simulink model "Electrical_System_2018b_obfs"  (R2019b)
settings: Solver=VariableStepAuto  StartTime=0.0  StopTime=5  RelTol=1e-3  AbsTol=1e-3  EnableMultiTasking=on
InitFcn:
  | Steady_State_Initialisation;
StopFcn:
  | %sscexplore(simlog);
  | %Logging
undefined symbols (not defined in the file): abrlhklxvp, aexgmhuedq, afmfmjnutg, afpphrjpnc, ahuxbyvruc, alarvljztt, amxnyqmnuw, aodrlwvqie, aolhmuplyq, aqpmguuqkg, auesgwirzl, aurophlnng, awamelrhru, ayfhvxflxn, azxkacuhqc, babszerikg, bawhdqanwq, bevoqecvei, bltjvqbchx, bmqsuewujl, bsmyqjfgnf, btvjbsmnve, bywgxqeadw, bziaduxaer, bzmcmdqocb, bzsvyvetat, ccsjnrbsih, cdvenygxwh, cedkrnslhx, cjheorclzs, cjrdshrtqx, ckhavyhcza, ckxewznhlz, cmrcgyiplk, conenicnws, cqkejbgjnn, csfnuwymhe, cunupkhwbh, cwzfvzuxxh, dcadmadufn, dcfponivnv, ddtrqjrhjn, dfhoxvkqas, dfrhtcwpne, dfvomcagjv, djijwylxea, dnmeqksrrm, dnzewbdkaa, dsqcykyxav, dtswwlttmm, ecumpidjtv, edegaywrct, ejjjsmnejc, eknqnehjdz, emvdetzouf, esxbqkbahr, etnkkbreiq, eunoiiiirw, ewewcuedir, fatkfxdhtc ... (+386)
libraries: fl_lib x802, ee_lib x362, fl_ps_legacy_lib x160, nesl_utility x85
(part 19 of 26)

== system Electrical_System_2018b_obfs/Redacted_1221/Redacted_7996/Redacted_7418/Redacted_4377/Redacted_6082/Redacted_5129 ==
  Redacted_1091 : ee_lib/Passive/Thermal/Thermal Resistor  R=xukkryhjsj K/W  T_specify=off  T_priority=None  T=tqiwxmipjo K  T_nominal_specify=off  T_nominal_unit=K  T_nominal_value=aelkngfktz  Q_specify=off  Q_priority=None  Q=uecypvqdqw W  Q_nominal_specify=off  Q_nominal_unit=W  Q_nominal_value=dfxrifobdg
      settings: SourceProductName=Simscape Electrical  SourceProductBaseCode=PS  InternalSimscapePortConfiguration="{\"Bottom\":[],\"Left\":[{\"id\":\"A\",\"label\":\"A\",\"type\":\"foundation.thermal.thermal\"}],\"Right\":[{\"id\":\"B\",\"label\":\"B\",\"type\":\"foundation.thermal.thermal\"}],\"Top\":[]}"
  Redacted_3516 : fl_lib/Electrical/Electrical Elements/Switch  R_closed=viaptkjwzx Ohm  G_open=spahjfgthv 1/Ohm  Threshold=dnzewbdkaa  i_specify=off  i_priority=None  i=solngxsjde A  i_nominal_specify=off  i_nominal_unit=A  i_nominal_value=kcgnlcicvg  v_specify=off  v_priority=None  v=pvqprocfho V  v_nominal_specify=off  v_nominal_unit=V  v_nominal_value=hvyevfetqr
      settings: SourceProductName=Simscape
  Redacted_4493 : ee_lib/Passive/Thermal/Thermal Resistor  R=vkzgeqezuu K/W  T_specify=off  T_priority=None  T=esxbqkbahr K  T_nominal_specify=off  T_nominal_unit=K  T_nominal_value=kzpyjzolsz  Q_specify=off  Q_priority=None  Q=zidswjyook W  Q_nominal_specify=off  Q_nominal_unit=W  Q_nominal_value=mpaskulynn
      settings: SourceProductName=Simscape Electrical  SourceProductBaseCode=PS  InternalSimscapePortConfiguration="{\"Bottom\":[],\"Left\":[{\"id\":\"A\",\"label\":\"A\",\"type\":\"foundation.thermal.thermal\"}],\"Right\":[{\"id\":\"B\",\"label\":\"B\",\"type\":\"foundation.thermal.thermal\"}],\"Top\":[]}"
  Redacted_5736 : ee_lib/Semiconductors & Converters/Diode  ModelType=scnymfcyan  Vf=usjfqlowdb V  Ron=jptklmkxco Ohm  Goff=ihriznynzt S  prmExp=aymyrnkeyq  I12=sbueuqiyue A  V12=xralefmnmn V  IS=aazejvtdlh A  ec=lidbrydnsj  I1=aanjbxmvih A  V1=csezzhepis V  RS=hlsmvzlbct Ohm  Tmeas=qwpxhludyc degC  N_series=ngscuduecf  N_parallel=mtvctablcr  Rz=kfmndsfqah Ohm  BV=bisvtzzlmp V  C_param=zzuhuqdxbf  CJ=dgdyeqdnad pF  CJ0=vviixrlmuw pF  VJ=erikpjzwum V  Mgrad=idrwctvgka  Vvec=okvogmauev V  Cvec=ltbtlumqgo pF  FC=hutzvqbjst  Q_param=tfxaxdyfov  iRM=mxcantmjiz A  iF=xjldnwmowj A  didt=knlmkgueiv A/us  trr_factor=zjmxnibovs  trr=xbruedlduk ns  Qrr=rqbcaonvzx s*uA  TT=sescozsnne ns  tau=onhgnodkyy ns  T_param=plqnodbxtj  IS_T2=gunyrtbbui A  I1_T2=kbaugpgxig A  V1_T2=pfkhkcpzef V  Tmeas2=tqjznseuwe degC  EG_param=derhodxtrf  EG=puioajbhgt eV  XTI_param=kgeisxvirz  XTI=ttohkaatoo  dBVdT=qouasokgzj V/K  Tdevice=hapcaufila degC  i_specify=off  i_priority=None  i=fhzvmzekzz A  i_nominal_specify=off  i_nominal_unit=A  i_nominal_value=gxbmpayvch  v_specify=off  v_priority=None  v=busuwkvnmf V  v_nominal_specify=off  v_nominal_unit=V  v_nominal_value=mquxmvisyo  i_capacitor_specify=off  i_capacitor_priority=None  i_capacitor=erdhqvbuqo A  i_capacitor_nominal_specify=off  i_capacitor_nominal_unit=A  i_capacitor_nominal_value=rircubgbtn  v_capacitor_specify=off  v_capacitor_priority=None  v_capacitor=ivjksolhtz V  v_capacitor_nominal_specify=off  v_capacitor_nominal_unit=V  v_capacitor_nominal_value=fbdfrcucsm  power_dissipated_specify=off  power_dissipated_priority=None  power_dissipated=kcgakdxjwx W  power_dissipated_nominal_specify=off  power_dissipated_nominal_unit=W  power_dissipated_nominal_value=hmtdzvxlgr  thermal_network_parameterization=ahnuexnajx  Rth=zqvcvxpppv K/W  Rth_Foster=pikijtguhr K/W  thermal_mass_parameterization=ebiijoiwcx  thermal_mass=xdfmtdtgha J/K  thermal_mass_Foster=alrgsxgqtc J/K  thermal_time_constant=vinydwuarm s  thermal_time_constant_Foster=gzkwvsvsmy s  thermal_mass_initial_temperatures=fpaqdrttzj degC
      settings: SourceProductName=Simscape Electrical  InternalSimscapePortConfiguration="{\"Bottom\":[],\"Left\":[{\"id\":\"p\",\"label\":\"\",\"type\":\"foundation.electrical.electrical\"},{\"id\":\"H\",\"label\":\"H\",\"type\":\"foundation.thermal.thermal\"}],\"Right\":[{\"id\":\"n\",\"label\":\"\",\"type\":\"foundation.electrical.electrical\"}],\"Top\":[]}"
  Redacted_5773 : ee_lib/Passive/Thermal/Thermal Resistor  R=pbykuyqcdd K/W  T_specify=off  T_priority=None  T=wxiejlvzgg K  T_nominal_specify=off  T_nominal_unit=K  T_nominal_value=mfkuttxvwe  Q_specify=off  Q_priority=None  Q=dxpebethas W  Q_nominal_specify=off  Q_nominal_unit=W  Q_nominal_value=tsjrjrjwno
      settings: SourceProductName=Simscape Electrical  SourceProductBaseCode=PS  InternalSimscapePortConfiguration="{\"Bottom\":[],\"Left\":[{\"id\":\"A\",\"label\":\"A\",\"type\":\"foundation.thermal.thermal\"}],\"Right\":[{\"id\":\"B\",\"label\":\"B\",\"type\":\"foundation.thermal.thermal\"}],\"Top\":[]}"
  Redacted_7843 : ee_lib/Semiconductors & Converters/Diode  ModelType=vfubjonbyz  Vf=ovhazgcrzk V  Ron=cvrskrmuqj Ohm  Goff=lhhixvbmqc S  prmExp=qjndrrcrwj  I12=gntvzaamtj A  V12=wuwbzbrrpp V  IS=hzdxbkvqke A  ec=lzufgtgbsv  I1=zjffddejik A  V1=ijrimogulp V  RS=ykiqzyljzc Ohm  Tmeas=htzzchmtfv degC  N_series=hvcvcsiwkf  N_parallel=xydvemqmiv  Rz=otkhgvieqq Ohm  BV=vuygfstuny V  C_param=cqqyubkwai  CJ=uoegdangwr pF  CJ0=plaiwchowh pF  VJ=yenohlnnoo V  Mgrad=eruhhyqxpf  Vvec=svfoknpnpk V  Cvec=zqjlotgxpq pF  FC=ortnyuwzrh  Q_param=zdzueyncpy  iRM=pnzdzmfzlv A  iF=jwwiykcvrz A  didt=hhhqlcepyp A/us  trr_factor=rznizglpmy  trr=swvxsytfmb ns  Qrr=rqufmcdvlt s*uA  TT=pecnigvizl ns  tau=ijpnmgbmsc ns  T_param=qpvjlpxidl  IS_T2=vidgyzqclm A  I1_T2=khiphkkgwk A  V1_T2=pizjjevhmz V  Tmeas2=qreuemgwhd degC  EG_param=ancfqgfkip  EG=ktrhgbakxp eV  XTI_param=brbgadfkca  XTI=ygqbsywepo  dBVdT=eqvegiauyi V/K  Tdevice=drlcvrgbtu degC  i_specify=off  i_priority=None  i=cqcsuzhiqx A  i_nominal_specify=off  i_nominal_unit=A  i_nominal_value=xlakfqcnpk  v_specify=off  v_priority=None  v=hictgeopsi V  v_nominal_specify=off  v_nominal_unit=V  v_nominal_value=ughojcypmy  i_capacitor_specify=off  i_capacitor_priority=None  i_capacitor=hpzqydefid A  i_capacitor_nominal_specify=off  i_capacitor_nominal_unit=A  i_capacitor_nominal_value=tcfiupnxkj  v_capacitor_specify=off  v_capacitor_priority=None  v_capacitor=jmshvmneul V  v_capacitor_nominal_specify=off  v_capacitor_nominal_unit=V  v_capacitor_nominal_value=gayfmkqmju  power_dissipated_specify=off  power_dissipated_priority=None  power_dissipated=mgodbrjsas W  power_dissipated_nominal_specify=off  power_dissipated_nominal_unit=W  power_dissipated_nominal_value=fxyfgqyyze  thermal_network_parameterization=fvnzxsjdmp  Rth=wolwfjnjmr K/W  Rth_Foster=qclpxpisnk K/W  thermal_mass_parameterization=gxtwroopga  thermal_mass=inuccawayp J/K  thermal_mass_Foster=fypkvhimoq J/K  thermal_time_constant=rqyvbrsfkk s  thermal_time_constant_Foster=gsviadgrbu s  thermal_mass_initial_temperatures=udushfwxsp degC
      settings: SourceProductName=Simscape Electrical  InternalSimscapePortConfiguration="{\"Bottom\":[],\"Left\":[{\"id\":\"p\",\"label\":\"\",\"type\":\"foundation.electrical.electrical\"},{\"id\":\"H\",\"label\":\"H\",\"type\":\"foundation.thermal.thermal\"}],\"Right\":[{\"id\":\"n\",\"label\":\"\",\"type\":\"foundation.electrical.electrical\"}],\"Top\":[]}"
  Redacted_9825 : fl_lib/Electrical/Electrical Elements/Switch  R_closed=khogqsphcc Ohm  G_open=bnklxlqulg 1/Ohm  Threshold=bzmcmdqocb  i_specify=off  i_priority=None  i=debufxhmtc A  i_nominal_specify=off  i_nominal_unit=A  i_nominal_value=aobdrgvdef  v_specify=off  v_priority=None  v=jvrbptenmb V  v_nominal_specify=off  v_nominal_unit=V  v_nominal_value=ocwrndnqbv
      settings: SourceProductName=Simscape
  Redacted_3870 : PMIOPort  Side=Left
  Redacted_9209 : PMIOPort  Port=2  Side=Left
  Redacted_7831 : PMIOPort  Port=3  Side=Right
  Redacted_499 : PMIOPort  Port=4  Side=Right
  Redacted_8800 : PMIOPort  Port=5  Side=Left
  Redacted_5226 : PMIOPort  Port=6  Side=Right
  connections:
  Redacted_7843/LConn2 -- Redacted_5773/LConn1
  Redacted_4493/RConn1 -- Redacted_8800/RConn1
  Redacted_499/RConn1 -- Redacted_3516/RConn2
  Redacted_9825/RConn1 -- Redacted_3516/RConn1 -- Redacted_5226/RConn1
  Redacted_1091/RConn1 -- Redacted_4493/LConn1 -- Redacted_5773/RConn1
  Redacted_3870/RConn1 -- Redacted_5736/RConn1
  Redacted_5736/LConn1 -- Redacted_9825/LConn1
  Redacted_7831/RConn1 -- Redacted_9825/RConn2
  Redacted_5736/LConn2 -- Redacted_1091/LConn1
  Redacted_7843/RConn1 -- Redacted_3516/LConn1
  Redacted_7843/LConn1 -- Redacted_9209/RConn1

== system Electrical_System_2018b_obfs/Redacted_1221/Redacted_7996/Redacted_7418/Redacted_4377/Redacted_6082/Redacted_538 ==
  Redacted_2474 : ee_lib/Passive/Thermal/Thermal Resistor  R=tlxbhmhcor K/W  T_specify=off  T_priority=None  T=glxcmexbqk K  T_nominal_specify=off  T_nominal_unit=K  T_nominal_value=rodxnpycsn  Q_specify=off  Q_priority=None  Q=qzyewlatml W  Q_nominal_specify=off  Q_nominal_unit=W  Q_nominal_value=gwgijjmpqo
      settings: SourceProductName=Simscape Electrical  SourceProductBaseCode=PS  InternalSimscapePortConfiguration="{\"Bottom\":[],\"Left\":[{\"id\":\"A\",\"label\":\"A\",\"type\":\"foundation.thermal.thermal\"}],\"Right\":[{\"id\":\"B\",\"label\":\"B\",\"type\":\"foundation.thermal.thermal\"}],\"Top\":[]}"
  Redacted_3959 : ee_lib/Semiconductors & Converters/Diode  ModelType=cvugfgmtfd  Vf=orelrxevia V  Ron=wxqqpmaddo Ohm  Goff=dngzjrqfwi S  prmExp=alwaagijeo  I12=ddqlkshwcb A  V12=xrkoiubeyy V  IS=xzqvhkoygc A  ec=mmbccpipxa  I1=ryagswhoik A  V1=yrovtgvtuv V  RS=cqohiqgcgo Ohm  Tmeas=hcgkqnpcsd degC  N_series=dhajyiyagh  N_parallel=twliypcbap  Rz=qwuyngymow Ohm  BV=nknpvrzxhu V  C_param=guvgzkombp  CJ=icairznadf pF  CJ0=mzqqqufhew pF  VJ=clgkkuemkj V  Mgrad=xeknterrpa  Vvec=epolkzdkro V  Cvec=ihzesxymmo pF  FC=renthmlyxq  Q_param=jdcgohbezp  iRM=qomoanohux A  iF=berhrdnhlf A  didt=nmtpqyoydb A/us  trr_factor=ellslhrnwb  trr=iwxktrkdlw ns  Qrr=lvsgqazssj s*uA  TT=djywuxkdvp ns  tau=dsvtaxiwkr ns  T_param=lkgbfzstdy  IS_T2=xxalayentz A  I1_T2=ouhmerbjva A  V1_T2=rsvjknjiop V  Tmeas2=gzwycyriyy degC  EG_param=ufydvnqgur  EG=awpclymgzc eV  XTI_param=hewsmdjtfl  XTI=uikenwfmwu  dBVdT=wnhlxqhthu V/K  Tdevice=oyhmqnvbqo degC  i_specify=off  i_priority=None  i=yuxtxukkqw A  i_nominal_specify=off  i_nominal_unit=A  i_nominal_value=tzdopizgpf  v_specify=off  v_priority=None  v=agbhwyzrpj V  v_nominal_specify=off  v_nominal_unit=V  v_nominal_value=ematotugcl  i_capacitor_specify=off  i_capacitor_priority=None  i_capacitor=xujmcaxirs A  i_capacitor_nominal_specify=off  i_capacitor_nominal_unit=A  i_capacitor_nominal_value=sdffyhujvl  v_capacitor_specify=off  v_capacitor_priority=None  v_capacitor=hxtlnoghbu V  v_capacitor_nominal_specify=off  v_capacitor_nominal_unit=V  v_capacitor_nominal_value=ulxhxpyrnl  power_dissipated_specify=off  power_dissipated_priority=None  power_dissipated=kejtoizjdb W  power_dissipated_nominal_specify=off  power_dissipated_nominal_unit=W  power_dissipated_nominal_value=zqnfawynfr  thermal_network_parameterization=drmprivida  Rth=ehoeehkluw K/W  Rth_Foster=rnfrlrqpxo K/W  thermal_mass_parameterization=qpxdavwohv  thermal_mass=dhvivgsoft J/K  thermal_mass_Foster=bbttosewnp J/K  thermal_time_constant=uruvbjugmy s  thermal_time_constant_Foster=vxxdggnndt s  thermal_mass_initial_temperatures=cxuqjhpxqo degC
      settings: SourceProductName=Simscape Electrical  InternalSimscapePortConfiguration="{\"Bottom\":[],\"Left\":[{\"id\":\"p\",\"label\":\"\",\"type\":\"foundation.electrical.electrical\"},{\"id\":\"H\",\"label\":\"H\",\"type\":\"foundation.thermal.thermal\"}],\"Right\":[{\"id\":\"n\",\"label\":\"\",\"type\":\"foundation.electrical.electrical\"}],\"Top\":[]}"
  Redacted_5204 : ee_lib/Semiconductors & Converters/Diode  ModelType=vhkfbcdxxi  Vf=hwocrhyzln V  Ron=nrejuoqraz Ohm  Goff=xoikkoxmpt S  prmExp=sshdgyqrid  I12=abapcaqksv A  V12=rcfonjwkhk V  IS=uxhycfgjjf A  ec=ccjnesusom  I1=dkqtptmenz A  V1=cwkuodtzyn V  RS=bilkvppmaj Ohm  Tmeas=yoefghiwnx degC  N_series=vbhwyhycfg  N_parallel=nkltgmwizt  Rz=hvsuszjqqa Ohm  BV=fiypzfmfcw V  C_param=oozhdefoba  CJ=sfgabkycgd pF  CJ0=fbfiajzyfi pF  VJ=oqefwzhbwp V  Mgrad=ljxgznyykq  Vvec=byqphrqwso V  Cvec=kiphagckdr pF  FC=cfchcpalde  Q_param=ctajamwbgf  iRM=zyzkgvwrwb A  iF=gzcqjdolru A  didt=ehosyigpsp A/us  trr_factor=yrcmqekjvi  trr=uxqgcepufe ns  Qrr=zdwkgjghcs s*uA  TT=gvqnwlgzwi ns  tau=vcapcgxzee ns  T_param=kdsbtpdywb  IS_T2=dytgzmkhng A  I1_T2=pmcdffsnwx A  V1_T2=yirsozpwmg V  Tmeas2=tadzfoaqtg degC  EG_param=lombnbdzaq  EG=syhamdjlbj eV  XTI_param=ujfmodxdji  XTI=pggidhagfw  dBVdT=jqycxgazic V/K  Tdevice=jamzfbwkuq degC  i_specify=off  i_priority=None  i=yrlsqtdcrj A  i_nominal_specify=off  i_nominal_unit=A  i_nominal_value=xvntcjckiw  v_specify=off  v_priority=None  v=jedxxskqdr V  v_nominal_specify=off  v_nominal_unit=V  v_nominal_value=havzscyyds  i_capacitor_specify=off  i_capacitor_priority=None  i_capacitor=tsjkkrkoym A  i_capacitor_nominal_specify=off  i_capacitor_nominal_unit=A  i_capacitor_nominal_value=gtnybtppoh  v_capacitor_specify=off  v_capacitor_priority=None  v_capacitor=kvzillyxwo V  v_capacitor_nominal_specify=off  v_capacitor_nominal_unit=V  v_capacitor_nominal_value=bigwvzuhqf  power_dissipated_specify=off  power_dissipated_priority=None  power_dissipated=hrgpyhajat W  power_dissipated_nominal_specify=off  power_dissipated_nominal_unit=W  power_dissipated_nominal_value=nzqvcegghq  thermal_network_parameterization=ptsabaosyw  Rth=gmkxekgtcr K/W  Rth_Foster=grktmnwzih K/W  thermal_mass_parameterization=bbnolzopgu  thermal_mass=mdlarzsjrd J/K  thermal_mass_Foster=bznhxpubkn J/K  thermal_time_constant=updbvvrtrk s  thermal_time_constant_Foster=thopflkoks s  thermal_mass_initial_temperatures=cwyiuwsawu degC
      settings: SourceProductName=Simscape Electrical  InternalSimscapePortConfiguration="{\"Bottom\":[],\"Left\":[{\"id\":\"p\",\"label\":\"\",\"type\":\"foundation.electrical.electrical\"},{\"id\":\"H\",\"label\":\"H\",\"type\":\"foundation.thermal.thermal\"}],\"Right\":[{\"id\":\"n\",\"label\":\"\",\"type\":\"foundation.electrical.electrical\"}],\"Top\":[]}"
  Redacted_5866 : ee_lib/Passive/Thermal/Thermal Resistor  R=yowuuinfal K/W  T_specify=off  T_priority=None  T=iyyjqewjxa K  T_nominal_specify=off  T_nominal_unit=K  T_nominal_value=cnwhogxdzi  Q_specify=off  Q_priority=None  Q=xatxitavcu W  Q_nominal_specify=off  Q_nominal_unit=W  Q_nominal_value=lovetezeec
      settings: SourceProductName=Simscape Electrical  SourceProductBaseCode=PS  InternalSimscapePortConfiguration="{\"Bottom\":[],\"Left\":[{\"id\":\"A\",\"label\":\"A\",\"type\":\"foundation.thermal.thermal\"}],\"Right\":[{\"id\":\"B\",\"label\":\"B\",\"type\":\"foundation.thermal.thermal\"}],\"Top\":[]}"
  Redacted_6815 : fl_lib/Electrical/Electrical Elements/Switch  R_closed=gkqjhdadlv Ohm  G_open=gspgtvvlfq 1/Ohm  Threshold=reaxmeylvl  i_specify=off  i_priority=None  i=jkwqanynmu A  i_nominal_specify=off  i_nominal_unit=A  i_nominal_value=retrrtohdd  v_specify=off  v_priority=None  v=bvhvmbtprm V  v_nominal_specify=off  v_nominal_unit=V  v_nominal_value=orfswznhsg
      settings: SourceProductName=Simscape
  Redacted_70 : ee_lib/Passive/Thermal/Thermal Resistor  R=radskbcesf K/W  T_specify=off  T_priority=None  T=pzbxgmpntj K  T_nominal_specify=off  T_nominal_unit=K  T_nominal_value=fxdfehzdjb  Q_specify=off  Q_priority=None  Q=wnpgpngqdb W  Q_nominal_specify=off  Q_nominal_unit=W  Q_nominal_value=mvvrjfvzjw
      settings: SourceProductName=Simscape Electrical  SourceProductBaseCode=PS  InternalSimscapePortConfiguration="{\"Bottom\":[],\"Left\":[{\"id\":\"A\",\"label\":\"A\",\"type\":\"foundation.thermal.thermal\"}],\"Right\":[{\"id\":\"B\",\"label\":\"B\",\"type\":\"foundation.thermal.thermal\"}],\"Top\":[]}"
  Redacted_8610 : fl_lib/Electrical/Electrical Elements/Switch  R_closed=ebbxigazsv Ohm  G_open=bymurvxztv 1/Ohm  Threshold=fatkfxdhtc  i_specify=off  i_priority=None  i=ooxbtdevdj A  i_nominal_specify=off  i_nominal_unit=A  i_nominal_value=vtutgwbqlf  v_specify=off  v_priority=None  v=bphxdwqdvi V  v_nominal_specify=off  v_nominal_unit=V  v_nominal_value=jxgusntfnc
      settings: SourceProductName=Simscape
  Redacted_1520 : PMIOPort  Side=Left
  Redacted_1920 : PMIOPort  Port=2  Side=Left
  Redacted_4965 : PMIOPort  Port=3  Side=Right
  Redacted_6828 : PMIOPort  Port=4  Side=Right
  Redacted_6082 : PMIOPort  Port=5  Side=Left
  Redacted_6905 : PMIOPort  Port=6  Side=Right
  connections:
  Redacted_3959/LConn1 -- Redacted_1920/RConn1
  Redacted_3959/RConn1 -- Redacted_6815/LConn1
  Redacted_5204/LConn2 -- Redacted_2474/LConn1
  Redacted_4965/RConn1 -- Redacted_8610/RConn2
  Redacted_5204/LConn1 -- Redacted_8610/LConn1
  Redacted_1520/RConn1 -- Redacted_5204/RConn1
  Redacted_5866/RConn1 -- Redacted_70/LConn1 -- Redacted_2474/RConn1
  Redacted_6905/RConn1 -- Redacted_6815/RConn1 -- Redacted_8610/RConn1
  Redacted_6828/RConn1 -- Redacted_6815/RConn2
  Redacted_70/RConn1 -- Redacted_6082/RConn1
  Redacted_3959/LConn2 -- Redacted_5866/LConn1

== system Electrical_System_2018b_obfs/Redacted_1221/Redacted_7996/Redacted_7418/Redacted_4377/Redacted_6082/Redacted_5550 ==
  Neutral_Negative : Subsystem  VariantControl=Variant1
  Positive_Neutral : Subsystem  VariantControl=Variant3
  Redacted_2952 : Subsystem  VariantControl=Variant2
  Redacted_6826 : PMIOPort  Side=Left
  Redacted_51 : PMIOPort  Port=2  Side=Left
  Redacted_9515 : PMIOPort  Port=3  Side=Left
  Redacted_375 : PMIOPort  Port=4  Side=Right
  Redacted_6304 : PMIOPort  Port=5  Side=Right

== system Electrical_System_2018b_obfs/Redacted_1221/Redacted_7996/Redacted_7418/Redacted_4377/Redacted_6082/Redacted_5711 ==
  Redacted_1131 : ee_lib/Semiconductors & Converters/Diode  ModelType=sgjcxllrwb  Vf=rezwarhnlc V  Ron=wbzpxlludr Ohm  Goff=tokjykannh S  prmExp=iwsikdclek  I12=ndxpqzjahu A  V12=oyqejwvxul V  IS=mveceiwvha A  ec=uuxcdrnxrh  I1=ofqmoxeuin A  V1=vhypwmzhjp V  RS=kpwjpdopvx Ohm  Tmeas=jbuqxwxids degC  N_series=xhtsnjlbqd  N_parallel=paajnctnwf  Rz=dwqreiwlqp Ohm  BV=yeooqkxzdk V  C_param=fuflydgeqt  CJ=ljpqbdycpo pF  CJ0=jbgrvpposm pF  VJ=ywlmgounuw V  Mgrad=zlqpkihwcd  Vvec=swnlxjsfea V  Cvec=tpransojiq pF  FC=teismtbows  Q_param=kzrgworrpy  iRM=enksfiblxd A  iF=bubyvkprkt A  didt=imidgzdgio A/us  trr_factor=kdehgjmswa  trr=ywtdexwfoq ns  Qrr=dyhowxpurl s*uA  TT=tdrpgsjpmg ns  tau=xwtxyhtqlh ns  T_param=kglbvnzolr  IS_T2=jjkoutammx A  I1_T2=hozxsnrmeo A  V1_T2=ojcyvtfvao V  Tmeas2=uzbilkqbml degC  EG_param=nqysccnfec  EG=ifucnavfam eV  XTI_param=wngxburzzp  XTI=ymmwmtduml  dBVdT=krekrcumku V/K  Tdevice=zrczwfcaxw degC  i_specify=off  i_priority=None  i=jssphwnvvg A  i_nominal_specify=off  i_nominal_unit=A  i_nominal_value=jibhoqemck  v_specify=off  v_priority=None  v=biwmugqnkj V  v_nominal_specify=off  v_nominal_unit=V  v_nominal_value=pllakottju  i_capacitor_specify=off  i_capacitor_priority=None  i_capacitor=gdasqvnftj A  i_capacitor_nominal_specify=off  i_capacitor_nominal_unit=A  i_capacitor_nominal_value=xlxqydjrzg  v_capacitor_specify=off  v_capacitor_priority=None  v_capacitor=jsbomwjeni V  v_capacitor_nominal_specify=off  v_capacitor_nominal_unit=V  v_capacitor_nominal_value=lbbdaqqoij  power_dissipated_specify=off  power_dissipated_priority=None  power_dissipated=ttqksqojpg W  power_dissipated_nominal_specify=off  power_dissipated_nominal_unit=W  power_dissipated_nominal_value=pktukgibmd  thermal_network_parameterization=ukdumittgs  Rth=xarbpsrvuf K/W  Rth_Foster=ehmdrospka K/W  thermal_mass_parameterization=igbepyqptu  thermal_mass=gcqxbhpikq J/K  thermal_mass_Foster=lennybeyrl J/K  thermal_time_constant=cyjedarpes s  thermal_time_constant_Foster=aczvdslxpi s  thermal_mass_initial_temperatures=vndblrhnsn degC
      settings: SourceProductName=Simscape Electrical  InternalSimscapePortConfiguration="{\"Bottom\":[],\"Left\":[{\"id\":\"p\",\"label\":\"\",\"type\":\"foundation.electrical.electrical\"},{\"id\":\"H\",\"label\":\"H\",\"type\":\"foundation.thermal.thermal\"}],\"Right\":[{\"id\":\"n\",\"label\":\"\",\"type\":\"foundation.electrical.electrical\"}],\"Top\":[]}"
  Redacted_2394 : fl_lib/Electrical/Electrical Elements/Switch  R_closed=softcbgoyi Ohm  G_open=mrgmmagxyi 1/Ohm  Threshold=afmfmjnutg  i_specify=off  i_priority=None  i=lmpryftbna A  i_nominal_specify=off  i_nominal_unit=A  i_nominal_value=rlcndthfub  v_specify=off  v_priority=None  v=qfybfotxik V  v_nominal_specify=off  v_nominal_unit=V  v_nominal_value=zyqcuaregq
      settings: SourceProductName=Simscape
  Redacted_3905 : ee_lib/Semiconductors & Converters/Diode  ModelType=nfeveyyrwk  Vf=zoxnipqvrl V  Ron=mtrtbspsae Ohm  Goff=dzrkkqnoys S  prmExp=ievifbrmqp  I12=mmnqlsbltn A  V12=iccotdqbos V  IS=mdvbhccktk A  ec=zvzvjmlaaq  I1=glkqrotric A  V1=yvlqfpnpng V  RS=nzwdscfish Ohm  Tmeas=nqkxyaekrd degC  N_series=nxssfyoknr  N_parallel=bahtqbhcpk  Rz=uddicyycvc Ohm  BV=lpfvklzlry V  C_param=fdmpjfrzqu  CJ=tlkmtlddns pF  CJ0=zlulxxuqkq pF  VJ=ehkmpglgid V  Mgrad=ttbwvlbyhc  Vvec=gsdwthuyom V  Cvec=lrvhhiuttc pF  FC=xzutmjviug  Q_param=qknxtjwyrl  iRM=prfitvseyr A  iF=kpkaitodiu A  didt=atkwyawqox A/us  trr_factor=utxssuipxd  trr=rrnoyzonvo ns  Qrr=dlavsnbofe s*uA  TT=ueprzvgvki ns  tau=jjxthajxlq ns  T_param=iixgioxeoz  IS_T2=wkxqlaxaiv A  I1_T2=zwqouuyrqp A  V1_T2=icvdtwdbib V  Tmeas2=quufchgzgc degC  EG_param=dwtsnaxksr  EG=acnxomkusk eV  XTI_param=vbeyylysip  XTI=xalaivvcmy  dBVdT=kxhlpasngh V/K  Tdevice=gzzizoikgr degC  i_specify=off  i_priority=None  i=tynowkxmpx A  i_nominal_specify=off  i_nominal_unit=A  i_nominal_value=uaygorgksr  v_specify=off  v_priority=None  v=tmrxmeyjrs V  v_nominal_specify=off  v_nominal_unit=V  v_nominal_value=bqcnnfwvrh  i_capacitor_specify=off  i_capacitor_priority=None  i_capacitor=imvbpaeqss A  i_capacitor_nominal_specify=off  i_capacitor_nominal_unit=A  i_capacitor_nominal_value=gybwnvfkmn  v_capacitor_specify=off  v_capacitor_priority=None  v_capacitor=igyzppqxtw V  v_capacitor_nominal_specify=off  v_capacitor_nominal_unit=V  v_capacitor_nominal_value=larocdhkvv  power_dissipated_specify=off  power_dissipated_priority=None  power_dissipated=lnzqmvpzim W  power_dissipated_nominal_specify=off  power_dissipated_nominal_unit=W  power_dissipated_nominal_value=spywrtkhsd  thermal_network_parameterization=hddxfofeyy  Rth=jullxwctpz K/W  Rth_Foster=nvhdmofkhg K/W  thermal_mass_parameterization=mkeqkoxjsc  thermal_mass=sxbbhkgscj J/K  thermal_mass_Foster=ktkpfefkzp J/K  thermal_time_constant=rzzrohaxsq s  thermal_time_constant_Foster=kpaqylfjiw s  thermal_mass_initial_temperatures=jazsdptkag degC
      settings: SourceProductName=Simscape Electrical  InternalSimscapePortConfiguration="{\"Bottom\":[],\"Left\":[{\"id\":\"p\",\"label\":\"\",\"type\":\"foundation.electrical.electrical\"},{\"id\":\"H\",\"label\":\"H\",\"type\":\"foundation.thermal.thermal\"}],\"Right\":[{\"id\":\"n\",\"label\":\"\",\"type\":\"foundation.electrical.electrical\"}],\"Top\":[]}"
  Redacted_5143 : ee_lib/Passive/Thermal/Thermal Resistor  R=ybijqqbkuj K/W  T_specify=off  T_priority=None  T=fxspchliwh K  T_nominal_specify=off  T_nominal_unit=K  T_nominal_value=ppuzbfrerj  Q_specify=off  Q_priority=None  Q=bynsukdflj W  Q_nominal_specify=off  Q_nominal_unit=W  Q_nominal_value=wzgdmbkzup
      settings: SourceProductName=Simscape Electrical  SourceProductBaseCode=PS  InternalSimscapePortConfiguration="{\"Bottom\":[],\"Left\":[{\"id\":\"A\",\"label\":\"A\",\"type\":\"foundation.thermal.thermal\"}],\"Right\":[{\"id\":\"B\",\"label\":\"B\",\"type\":\"foundation.thermal.thermal\"}],\"Top\":[]}"
  Redacted_5618 : fl_lib/Electrical/Electrical Elements/Switch  R_closed=kezykkwcel Ohm  G_open=kohltqvzvt 1/Ohm  Threshold=cdvenygxwh  i_specify=off  i_priority=None  i=hmjtisnfth A  i_nominal_specify=off  i_nominal_unit=A  i_nominal_value=nehnrbwlwu  v_specify=off  v_priority=None  v=yztjetatcm V  v_nominal_specify=off  v_nominal_unit=V  v_nominal_value=mbyxixcoyh
      settings: SourceProductName=Simscape
  Redacted_8133 : ee_lib/Passive/Thermal/Thermal Resistor  R=jumrqxyemk K/W  T_specify=off  T_priority=None  T=ohgunjtfhv K  T_nominal_specify=off  T_nominal_unit=K  T_nominal_value=iyidfkkalr  Q_specify=off  Q_priority=None  Q=paihpxggkf W  Q_nominal_specify=off  Q_nominal_unit=W  Q_nominal_value=epallypmhw
      settings: SourceProductName=Simscape Electrical  SourceProductBaseCode=PS  InternalSimscapePortConfiguration="{\"Bottom\":[],\"Left\":[{\"id\":\"A\",\"label\":\"A\",\"type\":\"foundation.thermal.thermal\"}],\"Right\":[{\"id\":\"B\",\"label\":\"B\",\"type\":\"foundation.thermal.thermal\"}],\"Top\":[]}"
  Redacted_9572 : ee_lib/Passive/Thermal/Thermal Resistor  R=ttoaasuswm K/W  T_specify=off  T_priority=None  T=nnfmlqeyqa K  T_nominal_specify=off  T_nominal_unit=K  T_nominal_value=fhorypsrxc  Q_specify=off  Q_priority=None  Q=ckuzftrrgq W  Q_nominal_specify=off  Q_nominal_unit=W  Q_nominal_value=fqmdqwvrwk
      settings: SourceProductName=Simscape Electrical  SourceProductBaseCode=PS  InternalSimscapePortConfiguration="{\"Bottom\":[],\"Left\":[{\"id\":\"A\",\"label\":\"A\",\"type\":\"foundation.thermal.thermal\"}],\"Right\":[{\"id\":\"B\",\"label\":\"B\",\"type\":\"foundation.thermal.thermal\"}],\"Top\":[]}"
  Redacted_4950 : PMIOPort  Side=Left
  Redacted_5258 : PMIOPort  Port=2  Side=Left
  Redacted_5892 : PMIOPort  Port=3  Side=Right
  Redacted_8207 : PMIOPort  Port=4  Side=Right
  Redacted_4180 : PMIOPort  Port=5  Side=Left
  Redacted_8951 : PMIOPort  Port=6  Side=Right
  connections:
  Redacted_3905/LConn2 -- Redacted_8133/LConn1
  Redacted_9572/RConn1 -- Redacted_4180/RConn1
  Redacted_8207/RConn1 -- Redacted_2394/RConn2
  Redacted_5618/RConn1 -- Redacted_2394/RConn1 -- Redacted_8951/RConn1
  Redacted_5143/RConn1 -- Redacted_9572/LConn1 -- Redacted_8133/RConn1
  Redacted_4950/RConn1 -- Redacted_1131/RConn1
  Redacted_1131/LConn1 -- Redacted_5618/LConn1
  Redacted_5892/RConn1 -- Redacted_5618/RConn2
  Redacted_1131/LConn2 -- Redacted_5143/LConn1
  Redacted_3905/RConn1 -- Redacted_2394/LConn1
  Redacted_3905/LConn1 -- Redacted_5258/RConn1

== system Electrical_System_2018b_obfs/Redacted_1221/Redacted_7996/Redacted_7418/Redacted_4377/Redacted_6082/Redacted_5713 ==
  Neutral_Negative : Subsystem  VariantControl=Variant1
  Positive_Neutral : Subsystem  VariantControl=Variant3
  Redacted_1184 : Subsystem  VariantControl=Variant2
  Redacted_6138 : PMIOPort  Side=Left
  Redacted_1431 : PMIOPort  Port=2  Side=Left
  Redacted_7946 : PMIOPort  Port=3  Side=Left
  Redacted_819 : PMIOPort  Port=4  Side=Right
  Redacted_4816 : PMIOPort  Port=5  Side=Right

== system Electrical_System_2018b_obfs/Redacted_1221/Redacted_7996/Redacted_7418/Redacted_4377/Redacted_6082/Redacted_5976 ==
  Neutral_Negative : Subsystem  VariantControl=Variant1
  Positive_Neutral : Subsystem  VariantControl=Variant3
  Redacted_5620 : Subsystem  VariantControl=Variant2
  Redacted_9241 : PMIOPort  Side=Left
  Redacted_5276 : PMIOPort  Port=2  Side=Left
  Redacted_2400 : PMIOPort  Port=3  Side=Left
  Redacted_5406 : PMIOPort  Port=4  Side=Right
  Redacted_1074 : PMIOPort  Port=5  Side=Right

== system Electrical_System_2018b_obfs/Redacted_1221/Redacted_7996/Redacted_7418/Redacted_4377/Redacted_6082/Redacted_6424 ==
  Neutral_Negative : Subsystem  VariantControl=Variant1
  Positive_Neutral : Subsystem  VariantControl=Variant3
  Redacted_7805 : Subsystem  VariantControl=Variant2
  Redacted_4582 : PMIOPort  Side=Left
  Redacted_1544 : PMIOPort  Port=2  Side=Left
  Redacted_1581 : PMIOPort  Port=3  Side=Left
  Redacted_1961 : PMIOPort  Port=4  Side=Right
  Redacted_7479 : PMIOPort  Port=5  Side=Right

== system Electrical_System_2018b_obfs/Redacted_1221/Redacted_7996/Redacted_7418/Redacted_4377/Redacted_6082/Redacted_6448 ==
  Redacted_2500 : ee_lib/Semiconductors & Converters/Diode  ModelType=efectnzfzk  Vf=jxmepmeowj V  Ron=qgxsnpyvap Ohm  Goff=yoppabgzkl S  prmExp=ubpcccmurz  I12=remshksgqe A  V12=lfyuowwnsp V  IS=kniawzssyt A  ec=shjfprvpho  I1=bqvkznozbx A  V1=kanhzjgbwy V  RS=xqskwtorcu Ohm  Tmeas=wkndwwjeju degC  N_series=oemgleyaog  N_parallel=rmwesacawc  Rz=uupgbnboph Ohm  BV=jmlshjudem V  C_param=ejznuqydbf  CJ=jnyvftnijl pF  CJ0=eocfcshsjc pF  VJ=rcqumjutus V  Mgrad=bpwyttzsav  Vvec=xmbkulzqwe V  Cvec=eqgbafiqja pF  FC=fzcbcscgmr  Q_param=hevnohlimn  iRM=fkisxhzojn A  iF=aecufenajy A  didt=wqayegsgya A/us  trr_factor=tyozkzrsye  trr=byygrqxzxs ns  Qrr=ecsprgxdxa s*uA  TT=estselsvjb ns  tau=lnvjuifvwe ns  T_param=jrnxklcvyp  IS_T2=pegzeyggnh A  I1_T2=dfmjfojaum A  V1_T2=dkkcmajvzi V  Tmeas2=mhkasfkmys degC  EG_param=agwssckltu  EG=rfaarmrbja eV  XTI_param=uxzupvrblg  XTI=ospysejegc  dBVdT=tootsfdmyr V/K  Tdevice=kzpnsiiwfr degC  i_specify=off  i_priority=None  i=eihvzvfrzd A  i_nominal_specify=off  i_nominal_unit=A  i_nominal_value=qmmhrurogd  v_specify=off  v_priority=None  v=hizlbruxfz V  v_nominal_specify=off  v_nominal_unit=V  v_nominal_value=ycpyizpqai  i_capacitor_specify=off  i_capacitor_priority=None  i_capacitor=zppifvcjba A  i_capacitor_nominal_specify=off  i_capacitor_nominal_unit=A  i_capacitor_nominal_value=fpmjfabdfd  v_capacitor_specify=off  v_capacitor_priority=None  v_capacitor=stollmyrll V  v_capacitor_nominal_specify=off  v_capacitor_nominal_unit=V  v_capacitor_nominal_value=kndonlhkoo  power_dissipated_specify=off  power_dissipated_priority=None  power_dissipated=btdavdcdiv W  power_dissipated_nominal_specify=off  power_dissipated_nominal_unit=W  power_dissipated_nominal_value=tkklgbzblp  thermal_network_parameterization=bljrklmcju  Rth=xhsqylwmob K/W  Rth_Foster=optpcutsoi K/W  thermal_mass_parameterization=ugcqtdtype  thermal_mass=jsyutsyost J/K  thermal_mass_Foster=twrmylwkjc J/K  thermal_time_constant=xnykkposzd s  thermal_time_constant_Foster=foiqukjmop s  thermal_mass_initial_temperatures=upiyseqegs degC
      settings: SourceProductName=Simscape Electrical  InternalSimscapePortConfiguration="{\"Bottom\":[],\"Left\":[{\"id\":\"p\",\"label\":\"\",\"type\":\"foundation.electrical.electrical\"},{\"id\":\"H\",\"label\":\"H\",\"type\":\"foundation.thermal.thermal\"}],\"Right\":[{\"id\":\"n\",\"label\":\"\",\"type\":\"foundation.electrical.electrical\"}],\"Top\":[]}"
  Redacted_359 : ee_lib/Semiconductors & Converters/Diode  ModelType=scvaiquffk  Vf=gurupglfta V  Ron=ftlaqddzvo Ohm  Goff=sbgfdffxay S  prmExp=ukcnmjtiae  I12=grbxogokac A  V12=wmzyrlvpsn V  IS=leyegtjcol A  ec=lwvjfwcdkf  I1=dljtokvayx A  V1=irawojoicp V  RS=axoqkcbxfn Ohm  Tmeas=aargryzkwo degC  N_series=kaksezvljy  N_parallel=xdnjyjftou  Rz=rcunxliptk Ohm  BV=hrrjansjso V  C_param=gklskhmoru  CJ=imyuobqtwk pF  CJ0=ewdqrpecjy pF  VJ=wfjksexohd V  Mgrad=jgqtcmmwqv  Vvec=aguvzvrglj V  Cvec=zssvjevjde pF  FC=oeclxcixjt  Q_param=xrpxrrdafl  iRM=bcqzohazjt A  iF=crytmcfhbt A  didt=sirllclhmt A/us  trr_factor=ziidcweruu  trr=wxebnnxvyt ns  Qrr=ausdiytbgo s*uA  TT=naewcxqzgl ns  tau=ctbkxtppav ns  T_param=kyxkskcyft  IS_T2=nshgzahsri A  I1_T2=xuvyuqjsme A  V1_T2=oltorpmvrx V  Tmeas2=gktjbxgqtx degC  EG_param=iwktfixgrg  EG=teimjuixxi eV  XTI_param=shpugjdkdk  XTI=yrdjcsecbk  dBVdT=volhbyrkkf V/K  Tdevice=ofrafibacf degC  i_specify=off  i_priority=None  i=qtezljymoi A  i_nominal_specify=off  i_nominal_unit=A  i_nominal_value=yxnhkqaqti  v_specify=off  v_priority=None  v=kbwxruyprv V  v_nominal_specify=off  v_nominal_unit=V  v_nominal_value=igljubvsuu  i_capacitor_specify=off  i_capacitor_priority=None  i_capacitor=mlyqgxdfvw A  i_capacitor_nominal_specify=off  i_capacitor_nominal_unit=A  i_capacitor_nominal_value=ujbiigzksz  v_capacitor_specify=off  v_capacitor_priority=None  v_capacitor=cojyhmmzxj V  v_capacitor_nominal_specify=off  v_capacitor_nominal_unit=V  v_capacitor_nominal_value=wujzjvntdo  power_dissipated_specify=off  power_dissipated_priority=None  power_dissipated=yxytktehoc W  power_dissipated_nominal_specify=off  power_dissipated_nominal_unit=W  power_dissipated_nominal_value=pjafufeysq  thermal_network_parameterization=tftjmfuyfl  Rth=qburaojkwt K/W  Rth_Foster=jtrsywfksp K/W  thermal_mass_parameterization=mpaelmbuic  thermal_mass=qbntcmqzdf J/K  thermal_mass_Foster=iddtfueyvm J/K  thermal_time_constant=ewlbqfzhqf s  thermal_time_constant_Foster=ircpsmtrsx s  thermal_mass_initial_temperatures=xmifunpacs degC
      settings: SourceProductName=Simscape Electrical  InternalSimscapePortConfiguration="{\"Bottom\":[],\"Left\":[{\"id\":\"p\",\"label\":\"\",\"type\":\"foundation.electrical.electrical\"},{\"id\":\"H\",\"label\":\"H\",\"type\":\"foundation.thermal.thermal\"}],\"Right\":[{\"id\":\"n\",\"label\":\"\",\"type\":\"foundation.electrical.electrical\"}],\"Top\":[]}"
  Redacted_4119 : fl_lib/Electrical/Electrical Elements/Switch  R_closed=nvzhbxdgzi Ohm  G_open=jocuywfdlu 1/Ohm  Threshold=ycxpvyjhxx  i_specify=off  i_priority=None  i=wyjfxhkfvg A  i_nominal_specify=off  i_nominal_unit=A  i_nominal_value=qhiybsolgq  v_specify=off  v_priority=None  v=qhliplaqbe V  v_nominal_specify=off  v_nominal_unit=V  v_nominal_value=dflzoctfhv
      settings: SourceProductName=Simscape
  Redacted_7045 : ee_lib/Passive/Thermal/Thermal Resistor  R=znufdvpgrp K/W  T_specify=off  T_priority=None  T=gjhwzpgvuf K  T_nominal_specify=off  T_nominal_unit=K  T_nominal_value=wamkuaqotp  Q_specify=off  Q_priority=None  Q=iffnecxdnj W  Q_nominal_specify=off  Q_nominal_unit=W  Q_nominal_value=vfrfuelbtd
      settings: SourceProductName=Simscape Electrical  SourceProductBaseCode=PS  InternalSimscapePortConfiguration="{\"Bottom\":[],\"Left\":[{\"id\":\"A\",\"label\":\"A\",\"type\":\"foundation.thermal.thermal\"}],\"Right\":[{\"id\":\"B\",\"label\":\"B\",\"type\":\"foundation.thermal.thermal\"}],\"Top\":[]}"
  Redacted_7113 : fl_lib/Electrical/Electrical Elements/Switch  R_closed=xpgttbnlcv Ohm  G_open=qgroafvezw 1/Ohm  Threshold=emvdetzouf  i_specify=off  i_priority=None  i=kqcxlhjixi A  i_nominal_specify=off  i_nominal_unit=A  i_nominal_value=serpbanljy  v_specify=off  v_priority=None  v=tquhywvxiq V  v_nominal_specify=off  v_nominal_unit=V  v_nominal_value=hqozyjemvy
      settings: SourceProductName=Simscape
  Redacted_7754 : ee_lib/Passive/Thermal/Thermal Resistor  R=pifghqliop K/W  T_specify=off  T_priority=None  T=liaimvkskv K  T_nominal_specify=off  T_nominal_unit=K  T_nominal_value=plbwxvjplh  Q_specify=off  Q_priority=None  Q=nitcggggrk W  Q_nominal_specify=off  Q_nominal_unit=W  Q_nominal_value=cufaoxszsm
      settings: SourceProductName=Simscape Electrical  SourceProductBaseCode=PS  InternalSimscapePortConfiguration="{\"Bottom\":[],\"Left\":[{\"id\":\"A\",\"label\":\"A\",\"type\":\"foundation.thermal.thermal\"}],\"Right\":[{\"id\":\"B\",\"label\":\"B\",\"type\":\"foundation.thermal.thermal\"}],\"Top\":[]}"
  Redacted_8069 : ee_lib/Passive/Thermal/Thermal Resistor  R=ykpjzexeck K/W  T_specify=off  T_priority=None  T=dcfponivnv K  T_nominal_specify=off  T_nominal_unit=K  T_nominal_value=qfeaychhrh  Q_specify=off  Q_priority=None  Q=umsrugkwnq W  Q_nominal_specify=off  Q_nominal_unit=W  Q_nominal_value=pcplguatyr
      settings: SourceProductName=Simscape Electrical  SourceProductBaseCode=PS  InternalSimscapePortConfiguration="{\"Bottom\":[],\"Left\":[{\"id\":\"A\",\"label\":\"A\",\"type\":\"foundation.thermal.thermal\"}],\"Right\":[{\"id\":\"B\",\"label\":\"B\",\"type\":\"foundation.thermal.thermal\"}],\"Top\":[]}"
  Redacted_9919 : PMIOPort  Side=Left
  Redacted_9600 : PMIOPort  Port=2  Side=Left
  Redacted_2456 : PMIOPort  Port=3  Side=Right
  Redacted_124 : PMIOPort  Port=4  Side=Right
  Redacted_8053 : PMIOPort  Port=5  Side=Left
  Redacted_4129 : PMIOPort  Port=6  Side=Right
  connections:
  Redacted_2500/LConn1 -- Redacted_9600/RConn1
  Redacted_2500/RConn1 -- Redacted_7113/LConn1
  Redacted_359/LConn2 -- Redacted_8069/LConn1
  Redacted_2456/RConn1 -- Redacted_4119/RConn2
  Redacted_359/LConn1 -- Redacted_4119/LConn1
  Redacted_9919/RConn1 -- Redacted_359/RConn1
  Redacted_7754/RConn1 -- Redacted_7045/LConn1 -- Redacted_8069/RConn1
  Redacted_4129/RConn1 -- Redacted_7113/RConn1 -- Redacted_4119/RConn1
  Redacted_124/RConn1 -- Redacted_7113/RConn2
  Redacted_7045/RConn1 -- Redacted_8053/RConn1
  Redacted_2500/LConn2 -- Redacted_7754/LConn1

== system Electrical_System_2018b_obfs/Redacted_1221/Redacted_7996/Redacted_7418/Redacted_4377/Redacted_6082/Redacted_6527 ==
  Redacted_1424 : fl_lib/Electrical/Electrical Elements/Switch  R_closed=uubemsahiq Ohm  G_open=ozvememgqv 1/Ohm  Threshold=hnjmvnuswb  i_specify=off  i_priority=None  i=itzyracony A  i_nominal_specify=off  i_nominal_unit=A  i_nominal_value=zqxgqfenru  v_specify=off  v_priority=None  v=wleqakrbwd V  v_nominal_specify=off  v_nominal_unit=V  v_nominal_value=wygbutdclo
      settings: SourceProductName=Simscape
  Redacted_1733 : ee_lib/Passive/Thermal/Thermal Resistor  R=qgzigcwvwq K/W  T_specify=off  T_priority=None  T=vssqyrasqs K  T_nominal_specify=off  T_nominal_unit=K  T_nominal_value=uvmszgxxre  Q_specify=off  Q_priority=None  Q=jpywnaxojq W  Q_nominal_specify=off  Q_nominal_unit=W  Q_nominal_value=kkwfnufnoo
      settings: SourceProductName=Simscape Electrical  SourceProductBaseCode=PS  InternalSimscapePortConfiguration="{\"Bottom\":[],\"Left\":[{\"id\":\"A\",\"label\":\"A\",\"type\":\"foundation.thermal.thermal\"}],\"Right\":[{\"id\":\"B\",\"label\":\"B\",\"type\":\"foundation.thermal.thermal\"}],\"Top\":[]}"
  Redacted_2307 : ee_lib/Semiconductors & Converters/Diode  ModelType=yygispdsap  Vf=ddgocjgltc V  Ron=fwvfaxzvnp Ohm  Goff=wfblsuugok S  prmExp=qxzndhluss  I12=sqshvrdiph A  V12=nfodczazgj V  IS=whobbihuku A  ec=abzzdvvrza  I1=rdkvkqhdyd A  V1=zvbmipings V  RS=jpbkbpprev Ohm  Tmeas=nwhqotdbur degC  N_series=tfmhjxhjrz  N_parallel=begksghsae  Rz=ruutgskgma Ohm  BV=knynobbzgk V  C_param=zzrudhbdpf  CJ=thqgethmmh pF  CJ0=bhxhuuybgj pF  VJ=wampydxduu V  Mgrad=eqjkzbyofp  Vvec=mmgcagzjpe V  Cvec=zawyetnrxx pF  FC=ahrrwotxui  Q_param=xzjdgflsym  iRM=agdsnvjalq A  iF=ffnfwdscvn A  didt=fdxjshyvxs A/us  trr_factor=mkmyfvfyes  trr=gacgpnqvgu ns  Qrr=bbyyevepig s*uA  TT=tucnxfnpvo ns  tau=jahxnwizgh ns  T_param=hcisegfjcv  IS_T2=cgermndsgq A  I1_T2=vpzanteidy A  V1_T2=ztiovvpyyv V  Tmeas2=wwduknfans degC  EG_param=nvxjhmwpig  EG=xogzvypibl eV  XTI_param=oyofysglfl  XTI=ktkazczzev  dBVdT=nymuoqofpc V/K  Tdevice=ytwxdnehpn degC  i_specify=off  i_priority=None  i=zbhtayrmow A  i_nominal_specify=off  i_nominal_unit=A  i_nominal_value=vbxoxffqhl  v_specify=off  v_priority=None  v=vksdaxyjuv V  v_nominal_specify=off  v_nominal_unit=V  v_nominal_value=kanmrfdloo  i_capacitor_specify=off  i_capacitor_priority=None  i_capacitor=axztnhmdly A  i_capacitor_nominal_specify=off  i_capacitor_nominal_unit=A  i_capacitor_nominal_value=zvchdgraoo  v_capacitor_specify=off  v_capacitor_priority=None  v_capacitor=pkrddeylhy V  v_capacitor_nominal_specify=off  v_capacitor_nominal_unit=V  v_capacitor_nominal_value=rrafgiklmt  power_dissipated_specify=off  power_dissipated_priority=None  power_dissipated=lxbrmovrpy W  power_dissipated_nominal_specify=off  power_dissipated_nominal_unit=W  power_dissipated_nominal_value=kpwlhtkzah  thermal_network_parameterization=ersljgwkre  Rth=dpxszekbmk K/W  Rth_Foster=sedshturqg K/W  thermal_mass_parameterization=hiobflsxct  thermal_mass=nanxcpyyrc J/K  thermal_mass_Foster=swbqkjbtue J/K  thermal_time_constant=ogdijojbab s  thermal_time_constant_Foster=poxzlosyls s  thermal_mass_initial_temperatures=vuabxoysws degC
      settings: SourceProductName=Simscape Electrical  InternalSimscapePortConfiguration="{\"Bottom\":[],\"Left\":[{\"id\":\"p\",\"label\":\"\",\"type\":\"foundation.electrical.electrical\"},{\"id\":\"H\",\"label\":\"H\",\"type\":\"foundation.thermal.thermal\"}],\"Right\":[{\"id\":\"n\",\"label\":\"\",\"type\":\"foundation.electrical.electrical\"}],\"Top\":[]}"
  Redacted_5471 : ee_lib/Semiconductors & Converters/Diode  ModelType=dylqyfrumb  Vf=djwjlavxgg V  Ron=wjabrhhflf Ohm  Goff=ozauqfzfha S  prmExp=ieadlxwboq  I12=vpknywidyi A  V12=kxgzcqifbg V  IS=vcjqsyxitp A  ec=xvocbgesta  I1=huqetrpfgu A  V1=iynwjgmjhg V  RS=epzvhgmnsg Ohm  Tmeas=xqcholenhs degC  N_series=akurbozukz  N_parallel=lpafsotiku  Rz=dksbfwxken Ohm  BV=fowtsskggn V  C_param=mnpnfxxqye  CJ=aicgqixsbh pF  CJ0=srulofhfse pF  VJ=ouozluioet V  Mgrad=gfwibmsyze  Vvec=zaumleognr V  Cvec=yumfhvbkfs pF  FC=oqewfcqqju  Q_param=dsbrgeddbn  iRM=oaxjisldwr A  iF=swkfaahtjk A  didt=lebtvikjdv A/us  trr_factor=aswjjjyqva  trr=lhjvtwshym ns  Qrr=juuqdlouyy s*uA  TT=hpxbjdimvz ns  tau=ejuitcqjpx ns  T_param=vtnictwnru  IS_T2=bwporktges A  I1_T2=epinzvdzxw A  V1_T2=vcakwitolb V  Tmeas2=ufhgbygray degC  EG_param=beqjzgrucc  EG=ysoejqncmm eV  XTI_param=ybyrlmockc  XTI=dftuoysnwu  dBVdT=nefgclzwgj V/K  Tdevice=mljvtbjnva degC  i_specify=off  i_priority=None  i=jwadwmquns A  i_nominal_specify=off  i_nominal_unit=A  i_nominal_value=gktrqjynpb  v_specify=off  v_priority=None  v=njcctfkoay V  v_nominal_specify=off  v_nominal_unit=V  v_nominal_value=jxheyghequ  i_capacitor_specify=off  i_capacitor_priority=None  i_capacitor=vmzfsoqwwu A  i_capacitor_nominal_specify=off  i_capacitor_nominal_unit=A  i_capacitor_nominal_value=qrccizfisq  v_capacitor_specify=off  v_capacitor_priority=None  v_capacitor=cxinpvqodn V  v_capacitor_nominal_specify=off  v_capacitor_nominal_unit=V  v_capacitor_nominal_value=apzgnesosv  power_dissipated_specify=off  power_dissipated_priority=None  power_dissipated=hgheroluap W  power_dissipated_nominal_specify=off  power_dissipated_nominal_unit=W  power_dissipated_nominal_value=phjvibdzdg  thermal_network_parameterization=givzvrzuan  Rth=iixviegddv K/W  Rth_Foster=gsdmkgpcqm K/W  thermal_mass_parameterization=zqrrqkoaxz  thermal_mass=fvqhopbxbu J/K  thermal_mass_Foster=hysvxqdxyw J/K  thermal_time_constant=yatkhnfcgl s  thermal_time_constant_Foster=ojtticlvlv s  thermal_mass_initial_temperatures=bmufljunea degC
      settings: SourceProductName=Simscape Electrical  InternalSimscapePortConfiguration="{\"Bottom\":[],\"Left\":[{\"id\":\"p\",\"label\":\"\",\"type\":\"foundation.electrical.electrical\"},{\"id\":\"H\",\"label\":\"H\",\"type\":\"foundation.thermal.thermal\"}],\"Right\":[{\"id\":\"n\",\"label\":\"\",\"type\":\"foundation.electrical.electrical\"}],\"Top\":[]}"
  Redacted_5989 : ee_lib/Passive/Thermal/Thermal Resistor  R=ytpfqnyozy K/W  T_specify=off  T_priority=None  T=rfkrxpivtt K  T_nominal_specify=off  T_nominal_unit=K  T_nominal_value=dvmqgiitak  Q_specify=off  Q_priority=None  Q=npjdipshuc W  Q_nominal_specify=off  Q_nominal_unit=W  Q_nominal_value=eerlcjerke
      settings: SourceProductName=Simscape Electrical  SourceProductBaseCode=PS  InternalSimscapePortConfiguration="{\"Bottom\":[],\"Left\":[{\"id\":\"A\",\"label\":\"A\",\"type\":\"foundation.thermal.thermal\"}],\"Right\":[{\"id\":\"B\",\"label\":\"B\",\"type\":\"foundation.thermal.thermal\"}],\"Top\":[]}"
  Redacted_6325 : fl_lib/Electrical/Electrical Elements/Switch  R_closed=arlniknull Ohm  G_open=hcbdoqshtz 1/Ohm  Threshold=qqftcuuewi  i_specify=off  i_priority=None  i=mltdghhuuz A  i_nominal_specify=off  i_nominal_unit=A  i_nominal_value=tzrqlrltkl  v_specify=off  v_priority=None  v=edsdzxsadv V  v_nominal_specify=off  v_nominal_unit=V  v_nominal_value=niuolmioqy
      settings: SourceProductName=Simscape
  Redacted_9115 : ee_lib/Passive/Thermal/Thermal Resistor  R=vruipktyzb K/W  T_specify=off  T_priority=None  T=qsufbscrtd K  T_nominal_specify=off  T_nominal_unit=K  T_nominal_value=grbzvqfklm  Q_specify=off  Q_priority=None  Q=htwqzangcg W  Q_nominal_specify=off  Q_nominal_unit=W  Q_nominal_value=uchgmkqgfm
      settings: SourceProductName=Simscape Electrical  SourceProductBaseCode=PS  InternalSimscapePortConfiguration="{\"Bottom\":[],\"Left\":[{\"id\":\"A\",\"label\":\"A\",\"type\":\"foundation.thermal.thermal\"}],\"Right\":[{\"id\":\"B\",\"label\":\"B\",\"type\":\"foundation.thermal.thermal\"}],\"Top\":[]}"
  Redacted_6828 : PMIOPort  Side=Left
  Redacted_6214 : PMIOPort  Port=2  Side=Left
  Redacted_7583 : PMIOPort  Port=3  Side=Right
  Redacted_3746 : PMIOPort  Port=4  Side=Right
  Redacted_1539 : PMIOPort  Port=5  Side=Left
  Redacted_7195 : PMIOPort  Port=6  Side=Right
  connections:
  Redacted_5471/LConn2 -- Redacted_5989/LConn1
  Redacted_1733/RConn1 -- Redacted_1539/RConn1
  Redacted_3746/RConn1 -- Redacted_6325/RConn2
  Redacted_1424/RConn1 -- Redacted_6325/RConn1 -- Redacted_7195/RConn1
  Redacted_9115/RConn1 -- Redacted_1733/LConn1 -- Redacted_5989/RConn1
  Redacted_6828/RConn1 -- Redacted_2307/RConn1
  Redacted_2307/LConn1 -- Redacted_1424/LConn1
  Redacted_7583/RConn1 -- Redacted_1424/RConn2
  Redacted_2307/LConn2 -- Redacted_9115/LConn1
  Redacted_5471/RConn1 -- Redacted_6325/LConn1
  Redacted_5471/LConn1 -- Redacted_6214/RConn1
